simulink model "task_4_subtask_1"  (R2023b)
settings: Solver=FixedStepDiscrete  StartTime=0.0  StopTime=(16+210)*16  RelTol=1e-3
libraries: commchan3 x1, dspstat3 x1
settings Model: Creator=bhalaaj  LastModifiedBy=AMEY THAKUR

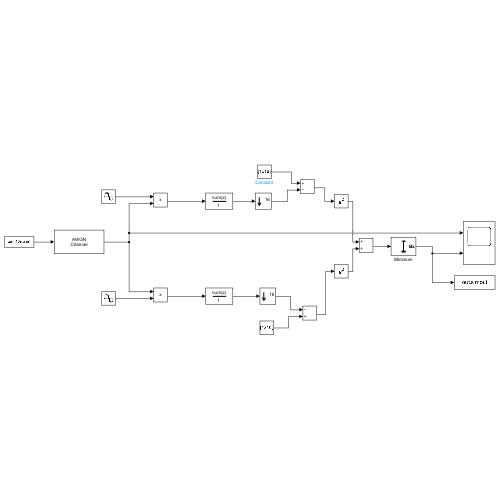
[thumbnail: Simulink's stored preview of the top-level diagram]
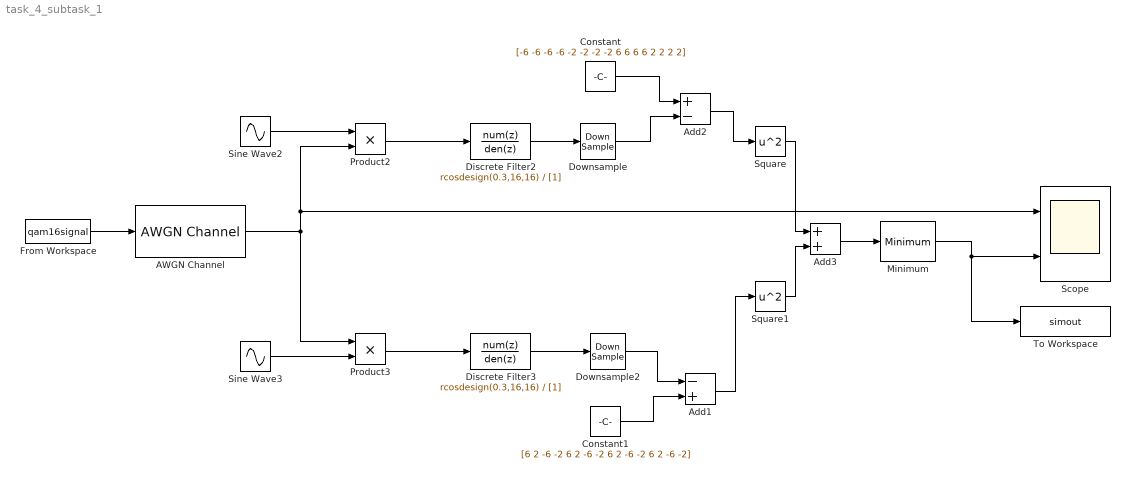
== system task_4_subtask_1 ==
  AWGN Channel : commchan3/AWGN Channel  LegacyMode=off  NoiseMethod="Signal to noise ratio  (Es/No)"  noiseMode="Signal to noise ratio  (SNR)"  EbNo=10  EsNo=40  SNR=10  BitsPerSymbol=1  SignalPower=1  SamplesPerSymbol=1  SymbolPeriod=1  VarianceSource=Parameter  Variance=1  RandomStream=mt19937ar with seed  Seed=110107589  SimulateUsing=Code generation
  Add1 : Sum  Inputs=-+
  Add2 : Sum  Inputs=+-
  Add3 : Sum
  Constant : Constant  Value=[-6 -6 -6 -6 -2 -2 -2 -2 6 6 6 6 2 2 2 2]
  Constant1 : Constant  Value=[6 2 -6 -2 6 2 -6 -2 6 2 -6 -2 6 2 -6 -2]
  Discrete Filter2 : DiscreteFilter  Numerator=rcosdesign(0.3,16,16)  Denominator=[1]
  Discrete Filter3 : DiscreteFilter  Numerator=rcosdesign(0.3,16,16)  Denominator=[1]
  Downsample : DownSample  N=16  RateOptions=Allow multirate processing  AllowArbitraryFixedInput=on
  Downsample2 : DownSample  N=16  RateOptions=Allow multirate processing  AllowArbitraryFixedInput=on
  From Workspace : FromWorkspace  VariableName=qam16signal  SampleTime=1
  Minimum : dspstat3/Minimum  operation=minimum  fcn=Index  indexBase=Zero  operateOver=Entire input  Dimension=1  InputProcessing=Columns as channels (frame based)  reset=None  roiEnable=off  roiType=Rectangles  roiPortion=Entire ROI  roiOutput=Individual statistics for each ROI  roiFlag=off  roundingMode=Floor  overflowMode=off
      settings: LibrarySourceBlock=dsphdlsupportstat/Minimum
  Product2 : Product
  Product3 : Product
  Scope : Scope  NumInputPorts=2
  Sine Wave2 : Sin  Amplitude=sqrt(2)  Frequency=0.5*pi  Phase=pi/2  SampleTime=1
  Sine Wave3 : Sin  Amplitude=-sqrt(2)  Frequency=0.5*pi  SampleTime=1
  Square : Math  Operator=square
  Square1 : Math  Operator=square
  To Workspace : ToWorkspace  VariableName=simout  SampleTime=-1
      settings: Save2DSignal=2-D array (concatenate along first dimension)
  wires:
  From Workspace/1 -> AWGN Channel/1
  Sine Wave2/1 -> Product2/1
  Sine Wave3/1 -> Product3/2
  AWGN Channel/1 -> Scope/1, Product2/2, Product3/1
  Product2/1 -> Discrete Filter2/1
  Product3/1 -> Discrete Filter3/1
  Discrete Filter2/1 -> Downsample/1
  Discrete Filter3/1 -> Downsample2/1
  Downsample/1 -> Add2/2
  Downsample2/1 -> Add1/1
  Add2/1 -> Square/1
  Add1/1 -> Square1/1
  Square/1 -> Add3/1
  Square1/1 -> Add3/2
  Add3/1 -> Minimum/1
  Minimum/1 -> To Workspace/1, Scope/2
  Constant/1 -> Add2/1
  Constant1/1 -> Add1/2
